simulink model "SSC17_QuanserPart3_SetupQuanser"  (R2014a)
settings: Solver=ode1  StartTime=0.0  StopTime=200  FixedStep=0.001  RelTol=1e-3
undefined symbols (not defined in the file or in its folder): HIL, qc_get_step_size
libraries: quarc_library x3
settings Model: SimulationMode=external  ExtModeTrigDuration=100000  Creator=MLevis  LastModifiedBy=ai15769
settings SolverCC: PositivePriorityOrder=on
settings DataIOCC: LimitDataPoints=off  SignalLoggingSaveFormat=ModelDataLogs
settings OptimizationCC: ExpressionDepthLimit=2147483647  InitFltsAndDblsToZero=on
settings DebuggingCC: SaveWithParameterizedLinksMsg=none  UnderspecifiedInitializationDetection=Classic  MultiTaskDSMMsg=warning  MultiTaskCondExecSysMsg=none  FcnCallInpInsideContextMsg=UseLocalSettings  StateNameClashWarn=warning  StrictBusMsg=None
settings RTWCC: SystemTargetFile=quarc_win64.tlc  TemplateMakefile=quarc_default_tmf  Description=QUARC Win64 Target  ProcessScript=quarc_win64_make_rtw_hook  IncludeERTFirstTime=on
settings STFCustomTargetCC: CPPClassGenCompliant=on
settings GRTTargetCC: ParMdlRefBuildCompliant=off  CompOptLevelCompliant=off  CombineOutputUpdateFcns=off  MatFileLogging=off  GRTInterface=on  ExtMode=on  ExtModeMexFile=quarc_comm

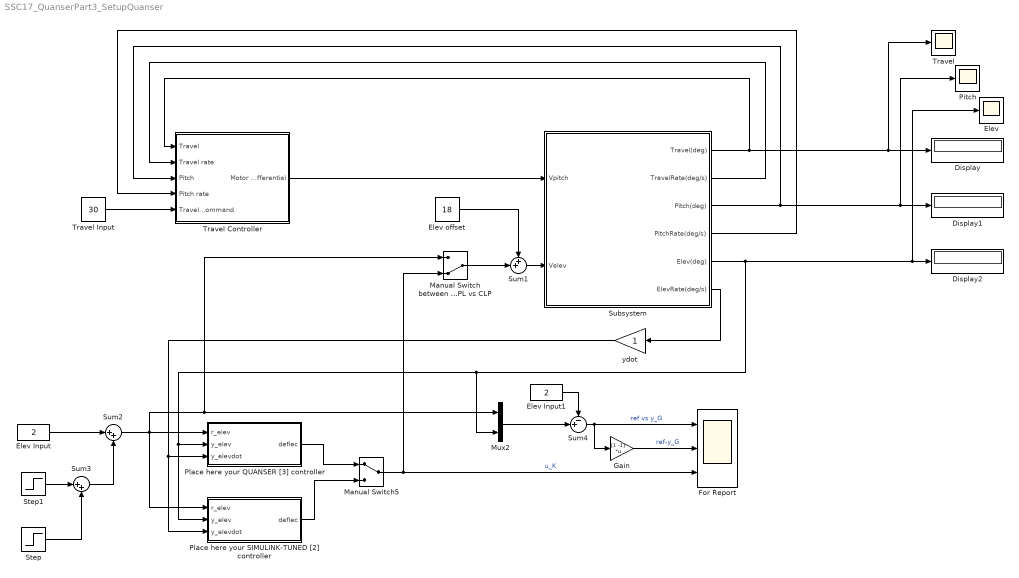
== system SSC17_QuanserPart3_SetupQuanser ==
  Display : Display
  Display1 : Display
  Display2 : Display
  Elev : Scope
      settings: TimeRange=100  YMin=-0  YMax=9  SaveName=elevData
  Elev Input : Constant  Value=2
  Elev Input1 : Constant  Value=2
  Elev offset : Constant  Value=18
  For Report : Scope  NumInputPorts=3
      settings: TimeRange=100  YMin=-3~-12~-22.5  YMax=12~3~2.5  SaveName=elevDataMINE
  Gain : Gain  Gain=[1 -1]  Multiplication=Matrix(K*u)
  Manual Switch between OPL vs CLP : ManualSwitch  CurrentSetting=0
  Manual Switch5 : ManualSwitch
  Mux2 : Mux  Inputs=2
  Pitch : Scope
      settings: TimeRange=100  YMin=-17.5  YMax=7.5  SaveName=pitchData
  Place here your QUANSER [3] controller : Subsystem
  Place here your SIMULINK-TUNED [2] controller : Subsystem
  Step : Step  Time=150  After=5  SampleTime=0
  Step1 : Step  Time=110  After=5  SampleTime=0
  Subsystem : Subsystem
  Sum1 : Sum  Inputs=++|
  Sum2 : Sum  Inputs=|++
  Sum3 : Sum  Inputs=|++
  Sum4 : Sum  Inputs=-+|
  Travel : Scope
      settings: TimeRange=100  YMin=0  YMax=45  SaveName=travelData
  Travel Controller : Subsystem
  Travel Input : Constant  Value=30
  ydot : Gain
  wires:
  Subsystem/1(Travel(deg)) -> Travel Controller/1(Travel), Travel/1, Display/1
  Subsystem/2(TravelRate(deg/s)) -> Travel Controller/2(Travel rate)
  Subsystem/3(Pitch(deg)) -> Travel Controller/3(Pitch), Pitch/1, Display1/1
  Subsystem/4(PitchRate(deg/s)) -> Travel Controller/4(Pitch rate)
  Subsystem/5(Elev(deg)) -> Mux2/2, Place here your SIMULINK-TUNED [2] controller/2(y_elev), Place here your QUANSER [3] controller/2(y_elev), Elev/1, Display2/1
  Travel Controller/1(Motor Differential) -> Subsystem/1(Vpitch)
  Sum1/1 -> Subsystem/2(Velev)
  Elev offset/1 -> Sum1/1
  Travel Input/1 -> Travel Controller/5(Travel Command)
  Subsystem/6(ElevRate(deg/s)) -> ydot/1
  Manual Switch between OPL vs CLP/1 -> Sum1/2
  Sum2/1 -> Place here your SIMULINK-TUNED [2] controller/1(r_elev), Place here your QUANSER [3] controller/1(r_elev), Manual Switch between OPL vs CLP/1, Mux2/1
  Manual Switch5/1 -> Manual Switch between OPL vs CLP/2, For Report/3  "u_K"
  ydot/1 -> Place here your SIMULINK-TUNED [2] controller/3(y_elevdot), Place here your QUANSER [3] controller/3(y_elevdot)
  Place here your QUANSER [3] controller/1(deflec) -> Manual Switch5/1
  Place here your SIMULINK-TUNED [2] controller/1(deflec) -> Manual Switch5/2
  Gain/1 -> For Report/2  "ref-y_G"
  Step1/1 -> Sum3/1
  Step/1 -> Sum3/2
  Sum3/1 -> Sum2/2
  Elev Input/1 -> Sum2/1
  Sum4/1 -> Gain/1, For Report/1  "ref vs y_G"
  Elev Input1/1 -> Sum4/1
  Mux2/1 -> Sum4/2

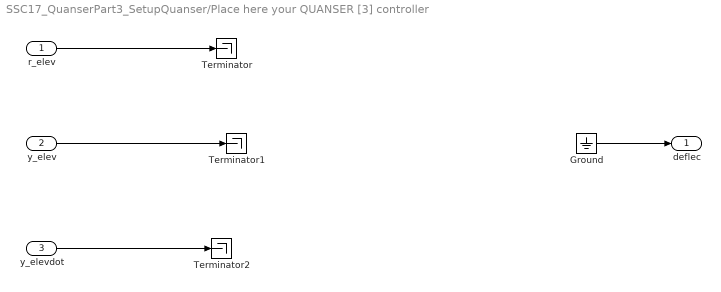
== system SSC17_QuanserPart3_SetupQuanser/Place here your QUANSER [3] controller ==
  r_elev : Inport
  y_elev : Inport  Port=2
  y_elevdot : Inport  Port=3
  Ground : Ground
  Terminator : Terminator
  Terminator1 : Terminator
  Terminator2 : Terminator
  deflec : Outport
  wires:
  r_elev/1 -> Terminator/1
  Ground/1 -> deflec/1
  y_elev/1 -> Terminator1/1
  y_elevdot/1 -> Terminator2/1

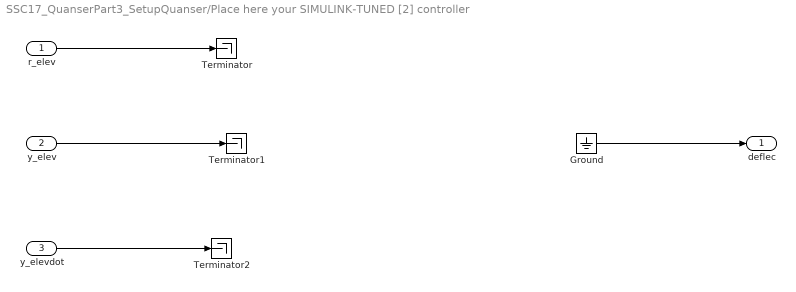
== system SSC17_QuanserPart3_SetupQuanser/Place here your SIMULINK-TUNED [2] controller ==
  r_elev : Inport
  y_elev : Inport  Port=2
  y_elevdot : Inport  Port=3
  Ground : Ground
  Terminator : Terminator
  Terminator1 : Terminator
  Terminator2 : Terminator
  deflec : Outport
  wires:
  r_elev/1 -> Terminator/1
  y_elev/1 -> Terminator1/1
  y_elevdot/1 -> Terminator2/1
  Ground/1 -> deflec/1

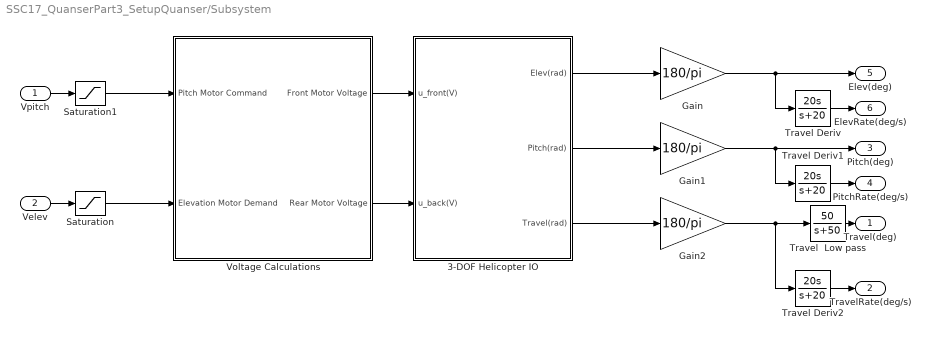
== system SSC17_QuanserPart3_SetupQuanser/Subsystem ==
  Vpitch : Inport
  Velev : Inport  Port=2
  3-DOF Helicopter IO : Subsystem
  Gain : Gain  Gain=180/pi
  Gain1 : Gain  Gain=180/pi
  Gain2 : Gain  Gain=180/pi
  Saturation : Saturate  UpperLimit=25  LowerLimit=-25
  Saturation1 : Saturate  UpperLimit=25  LowerLimit=-25
  Travel  Low pass : TransferFcn  Numerator=[50]  Denominator=[1 50]
  Travel Deriv : TransferFcn  Numerator=[20 0]  Denominator=[1 20]
  Travel Deriv1 : TransferFcn  Numerator=[20 0]  Denominator=[1 20]
  Travel Deriv2 : TransferFcn  Numerator=[20 0]  Denominator=[1 20]
  Voltage Calculations : Subsystem
  Travel(deg) : Outport
  TravelRate(deg/s) : Outport  Port=2
  Pitch(deg) : Outport  Port=3
  PitchRate(deg/s) : Outport  Port=4
  Elev(deg) : Outport  Port=5
  ElevRate(deg/s) : Outport  Port=6
  wires:
  3-DOF Helicopter IO/3(Travel(rad)) -> Gain2/1
  3-DOF Helicopter IO/2(Pitch(rad)) -> Gain1/1
  3-DOF Helicopter IO/1(Elev(rad)) -> Gain/1
  Gain/1 -> Travel Deriv/1, Elev(deg)/1
  Gain1/1 -> Travel Deriv1/1, Pitch(deg)/1
  Gain2/1 -> Travel Deriv2/1, Travel  Low pass/1
  Saturation/1 -> Voltage Calculations/2(Elevation Motor Demand)
  Voltage Calculations/2(Rear Motor Voltage) -> 3-DOF Helicopter IO/2(u_back(V))
  Voltage Calculations/1(Front Motor Voltage) -> 3-DOF Helicopter IO/1(u_front(V))
  Saturation1/1 -> Voltage Calculations/1(Pitch Motor Command)
  Vpitch/1 -> Saturation1/1
  Travel Deriv/1 -> ElevRate(deg/s)/1
  Travel Deriv1/1 -> PitchRate(deg/s)/1
  Velev/1 -> Saturation/1
  Travel  Low pass/1 -> Travel(deg)/1
  Travel Deriv2/1 -> TravelRate(deg/s)/1

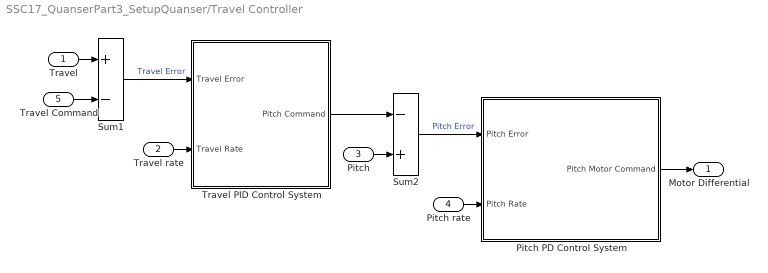
== system SSC17_QuanserPart3_SetupQuanser/Travel Controller ==
  Travel : Inport
  Travel rate : Inport  Port=2
  Pitch : Inport  Port=3
  Pitch rate : Inport  Port=4
  Travel Command : Inport  Port=5
  Pitch PD Control System : Subsystem
  Sum1 : Sum  Inputs=+-  SaturateOnIntegerOverflow=on  InputSameDT=on  OutDataTypeStr=Inherit: Same as first input
  Sum2 : Sum  Inputs=-+  SaturateOnIntegerOverflow=on  InputSameDT=on  OutDataTypeStr=Inherit: Same as first input
  Travel PID Control System : Subsystem
  Motor Differential : Outport
  wires:
  Travel/1 -> Sum1/1
  Travel PID Control System/1(Pitch Command) -> Sum2/1
  Pitch/1 -> Sum2/2
  Pitch rate/1 -> Pitch PD Control System/2(Pitch Rate)
  Sum2/1 -> Pitch PD Control System/1(Pitch Error)  "Pitch Error"
  Travel rate/1 -> Travel PID Control System/2(Travel Rate)
  Sum1/1 -> Travel PID Control System/1(Travel Error)  "Travel Error"
  Travel Command/1 -> Sum1/2
  Pitch PD Control System/1(Pitch Motor Command) -> Motor Differential/1

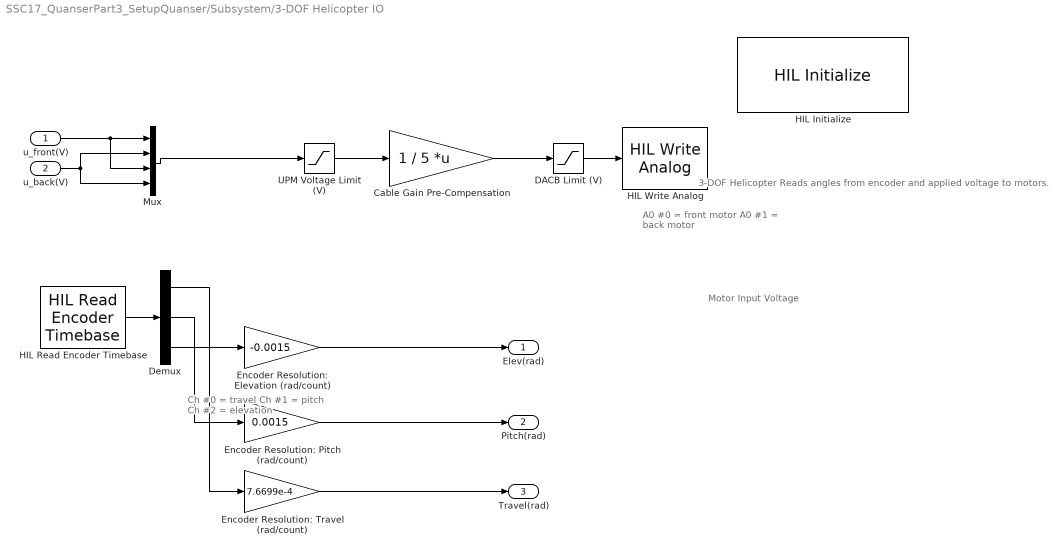
== system SSC17_QuanserPart3_SetupQuanser/Subsystem/3-DOF Helicopter IO ==
  note: A0 #0 = front motor
      | A0 #1 = back motor
  note: Motor Input Voltage
  note: 3-DOF Helicopter
      | Reads angles from encoder and applied voltage to motors.
  note: Ch #0 = travel
      | Ch #1 = pitch
      | Ch #2 = elevation
  u_front(V) : Inport
  u_back(V) : Inport  Port=2
  Cable Gain Pre-Compensation : Gain  Gain=1 / 5  Multiplication=Matrix(K*u)  SaturateOnIntegerOverflow=on  OutDataTypeStr=Inherit: Same as input  ParamDataTypeStr=Inherit: Same as input
  DACB Limit (V) : Saturate  UpperLimit=10  LowerLimit=-10
  Demux : Demux  Outputs=3
  Encoder Resolution: Elevation (rad/count) : Gain  Gain=-0.0015
  Encoder Resolution: Pitch (rad/count) : Gain  Gain=0.0015
  Encoder Resolution: Travel (rad/count) : Gain  Gain=7.6699e-4
  HIL Initialize : quarc_library/Data Acquisition/Generic/Configuration/HIL Initialize  object_name=HIL-1  board_type=q4  board_number=0  exclusive=off  active=on  hardware_clocks=[0:1]  clock_modes=[0 0]  initial_clock_frequencies=[]  set_clock_params_at_start=on  set_clock_params_at_switch_in=off  set_clock_frequencies_at_start=off  set_clock_frequencies_at_switch_in=off  analog_input_channels=[0:3]  analog_input_maximums=10  analog_input_minimums=-10  set_analog_input_params_at_start=off  set_analog_input_params_at_switch_in=off  analog_output_channels=[0:3]  analog_output_maximums=[10]  analog_output_minimums=[-10]  initial_analog_outputs=[0]  final_analog_outputs=[0]  watchdog_analog_outputs=0  set_analog_output_params_at_start=on  set_analog_output_params_at_switch_in=off  set_analog_outputs_at_start=on  set_analog_outputs_at_switch_in=off  set_analog_outputs_at_terminate=on  set_analog_outputs_at_switch_out=off  set_analog_outputs_on_watchdog=off  digital_input_channels=[]  digital_output_channels=[]  digital_output_configuration=[]  initial_digital_outputs=[1]  final_digital_outputs=[1]  watchdog_digital_outputs=[2]  set_digital_output_params_at_start=off  set_digital_output_params_at_switch_in=off  set_digital_outputs_at_start=on  set_digital_outputs_at_switch_in=off  set_digital_outputs_at_terminate=on  set_digital_outputs_at_switch_out=off  set_digital_outputs_on_watchdog=off  encoder_channels=[0:3]  quadrature=[4]  encoder_filter_frequency=(1/60e-9)/1  initial_encoder_counts=[0]  set_encoder_params_at_start=on  set_encoder_params_at_switch_in=off  set_encoder_counts_at_start=on  set_encoder_counts_at_switch_in=off  pwm_channels=[]  pwm_modes=[0]  pwm_frequency=(1/60e-9)/1024  pwm_configuration=[]  pwm_alignment=[]  pwm_polarity=[]  pwm_leading_deadband=[]  pwm_trailing_deadband=[]  initial_pwm_outputs=[0]  final_pwm_outputs=[0]  watchdog_pwm_outputs=[]  set_pwm_params_at_start=on  set_pwm_params_at_switch_in=off  set_pwm_outputs_at_start=on  set_pwm_outputs_at_switch_in=off  set_pwm_outputs_at_terminate=on  set_pwm_outputs_at_switch_out=off  set_pwm_outputs_on_watchdog=off  other_output_channels=[]  initial_other_outputs=[]  final_other_outputs=[]  watchdog_other_outputs=[]  set_other_outputs_at_start=off  set_other_outputs_at_switch_in=off  set_other_outputs_at_terminate=off  set_other_outputs_at_switch_out=off  set_other_outputs_on_watchdog=off
  HIL Read Encoder Timebase : quarc_library/Data Acquisition/Generic/Timebases/HIL Read Encoder Timebase  object_name=HIL-1  clock=0  channels=[0:2]  samples_in_buffer=max(ceil(1/qc_get_step_size), 1)  active=on  vector_output=on  data_type_mode=Inherit via back propagation  data_type=double
  HIL Write Analog : quarc_library/Data Acquisition/Generic/Immediate I//O/HIL Write Analog  object_name=HIL-1  channels=[0,1,2,3]  sample_time=-1  active=off  vector_input=on
  Mux : Mux
  UPM Voltage Limit (V) : Saturate  UpperLimit=24  LowerLimit=-24
  Elev(rad) : Outport
  Pitch(rad) : Outport  Port=2
  Travel(rad) : Outport  Port=3
  wires:
  HIL Read Encoder Timebase/1 -> Demux/1
  Encoder Resolution: Elevation (rad/count)/1 -> Elev(rad)/1
  Cable Gain Pre-Compensation/1 -> DACB Limit (V)/1
  UPM Voltage Limit (V)/1 -> Cable Gain Pre-Compensation/1
  DACB Limit (V)/1 -> HIL Write Analog/1
  Demux/3 -> Encoder Resolution: Elevation (rad/count)/1
  Demux/1 -> Encoder Resolution: Travel (rad/count)/1
  Demux/2 -> Encoder Resolution: Pitch (rad/count)/1
  Encoder Resolution: Travel (rad/count)/1 -> Travel(rad)/1
  Encoder Resolution: Pitch (rad/count)/1 -> Pitch(rad)/1
  Mux/1 -> UPM Voltage Limit (V)/1
  u_front(V)/1 -> Mux/1, Mux/3
  u_back(V)/1 -> Mux/2, Mux/4

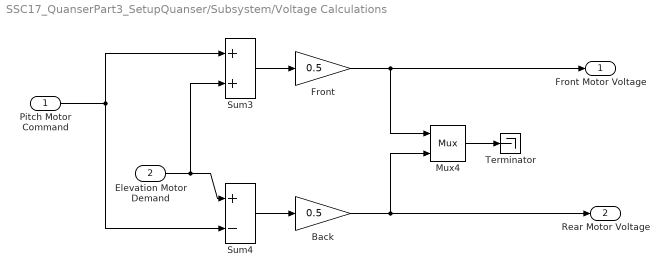
== system SSC17_QuanserPart3_SetupQuanser/Subsystem/Voltage Calculations ==
  Pitch Motor Command : Inport
  Elevation Motor Demand : Inport  Port=2
  Back : Gain  Gain=0.5  SaturateOnIntegerOverflow=on  OutDataTypeStr=Inherit: Same as input  ParamDataTypeStr=Inherit: Same as input
  Front : Gain  Gain=0.5  SaturateOnIntegerOverflow=on  OutDataTypeStr=Inherit: Same as input  ParamDataTypeStr=Inherit: Same as input
  Mux4 : Mux  Inputs=2
  Sum3 : Sum  SaturateOnIntegerOverflow=on  InputSameDT=on  OutDataTypeStr=Inherit: Same as first input
  Sum4 : Sum  Inputs=+-  SaturateOnIntegerOverflow=on  InputSameDT=on  OutDataTypeStr=Inherit: Same as first input
  Terminator : Terminator
  Front Motor Voltage : Outport
  Rear Motor Voltage : Outport  Port=2
  wires:
  Pitch Motor Command/1 -> Sum4/2, Sum3/1
  Sum3/1 -> Front/1
  Sum4/1 -> Back/1
  Elevation Motor Demand/1 -> Sum4/1, Sum3/2
  Mux4/1 -> Terminator/1
  Front/1 -> Mux4/1, Front Motor Voltage/1
  Back/1 -> Mux4/2, Rear Motor Voltage/1

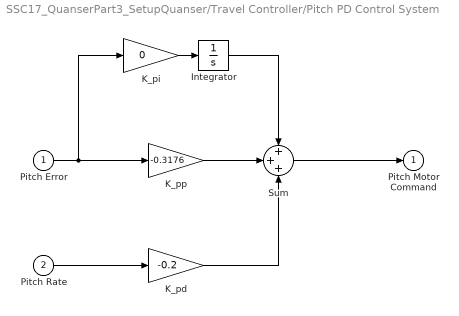
== system SSC17_QuanserPart3_SetupQuanser/Travel Controller/Pitch PD Control System ==
  Pitch Error : Inport
  Pitch Rate : Inport  Port=2
  Integrator : Integrator  LimitOutput=on  UpperSaturationLimit=5  LowerSaturationLimit=-5
  K_pd : Gain  Gain=-0.2  SaturateOnIntegerOverflow=on  OutDataTypeStr=Inherit: Same as input  ParamDataTypeStr=Inherit: Same as input
  K_pi : Gain  Gain=0  SaturateOnIntegerOverflow=on  OutDataTypeStr=Inherit: Same as input  ParamDataTypeStr=Inherit: Same as input
  K_pp : Gain  Gain=-0.3176  SaturateOnIntegerOverflow=on  OutDataTypeStr=Inherit: Same as input  ParamDataTypeStr=Inherit: Same as input
  Sum : Sum  Inputs=+++  SaturateOnIntegerOverflow=on  InputSameDT=on  OutDataTypeStr=Inherit: Same as first input
  Pitch Motor Command : Outport  InitialOutput=0
  wires:
  K_pi/1 -> Integrator/1
  Integrator/1 -> Sum/1
  Sum/1 -> Pitch Motor Command/1
  Pitch Rate/1 -> K_pd/1
  K_pd/1 -> Sum/3
  K_pp/1 -> Sum/2
  Pitch Error/1 -> K_pp/1, K_pi/1

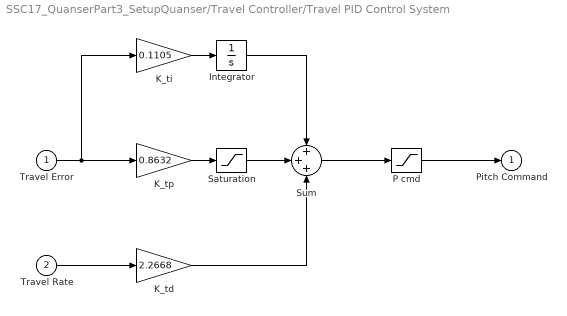
== system SSC17_QuanserPart3_SetupQuanser/Travel Controller/Travel PID Control System ==
  Travel Error : Inport
  Travel Rate : Inport  Port=2
  Integrator : Integrator  LimitOutput=on  UpperSaturationLimit=90  LowerSaturationLimit=-90
  K_td : Gain  Gain=2.2668  SaturateOnIntegerOverflow=on  OutDataTypeStr=Inherit: Same as input  ParamDataTypeStr=Inherit: Same as input
  K_ti : Gain  Gain=0.1105  SaturateOnIntegerOverflow=on  OutDataTypeStr=Inherit: Same as input  ParamDataTypeStr=Inherit: Same as input
  K_tp : Gain  Gain=0.8632  SaturateOnIntegerOverflow=on  OutDataTypeStr=Inherit: Same as input  ParamDataTypeStr=Inherit: Same as input
  P cmd : Saturate  UpperLimit=40  LowerLimit=-40
  Saturation : Saturate  UpperLimit=90  LowerLimit=-90
  Sum : Sum  Inputs=+++  SaturateOnIntegerOverflow=on  InputSameDT=on  OutDataTypeStr=Inherit: Same as first input
  Pitch Command : Outport  InitialOutput=0
  wires:
  Travel Error/1 -> K_ti/1, K_tp/1
  Travel Rate/1 -> K_td/1
  K_ti/1 -> Integrator/1
  K_tp/1 -> Saturation/1
  Saturation/1 -> Sum/2
  Sum/1 -> P cmd/1
  P cmd/1 -> Pitch Command/1
  Integrator/1 -> Sum/1
  K_td/1 -> Sum/3
